simulink model "case5new"  (Simulink 5.0)
settings: Solver=FixedStepDiscrete  SolverMode=SingleTasking  StartTime=0.0  StopTime=1  FixedStep=Ts  RelTol=1e-3  AbsTol=1e-2
PreLoadFcn:
  | assignin('base','Ts',[50e-6])
InitFcn:
  | powericon('psbinitsys',bdroot);
undefined symbols (not defined in the file): D1, Delta, gcbh, powericon, Ts
libraries: powerlib2 x65, powerlib_extras x5
settings Model: Creator=sybille  LastModifiedBy=gnedin pa  ExtModeTrigMode=oneshot  ExtModeArmWhenConnect=off  SaveTime=off  LimitDataPoints=off  UnconnectedInputMsg=none  UnconnectedOutputMsg=none  BlockReductionOpt=off  BooleanDataType=off

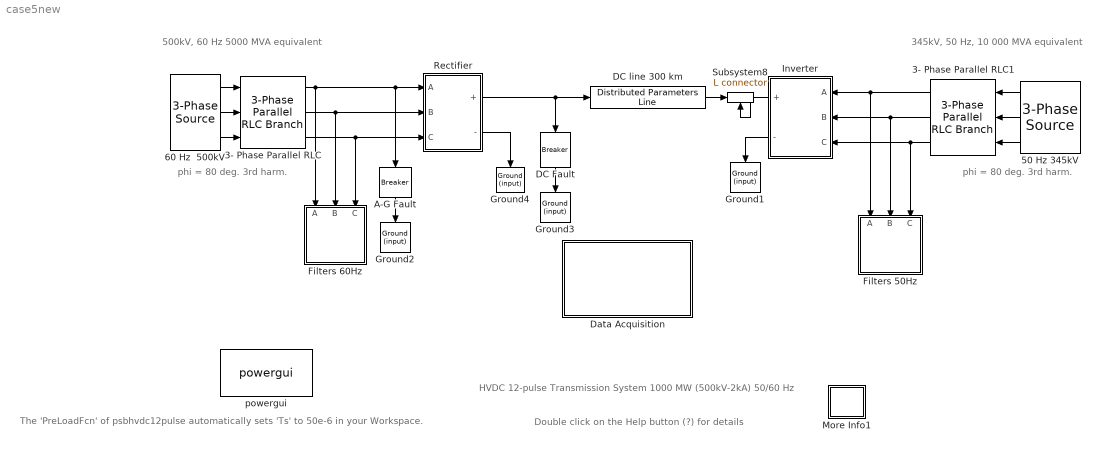
== system case5new ==
  note: phi = 80 deg. 3rd harm.
  note: The 'PreLoadFcn' of psbhvdc12pulse
      | automatically sets 'Ts' to 50e-6 in your Workspace.
  note: Double click on the Help button (?) for details
  note: HVDC 12-pulse Transmission System
      | 1000 MW (500kV-2kA)   50/60 Hz
  note: 500kV, 60 Hz
      |  5000 MVA equivalent
  note: 345kV, 50 Hz,
      | 10 000 MVA equivalent
  note: phi = 80 deg. 3rd harm.
  " 50 Hz 345kV  " : powerlib2/Electrical Sources/3-Phase Source  Tag=PoWeRsYsTeMbLoCk  Orientation=left  V=345e3  Phi=0  F=50  InternalConnection=Yg  RLoff=off  R=0  L=28.0e-3  Psc=0  Vbase=0  XRratio=0  PSBOutputType=111
  " 60 Hz  500kV" : powerlib2/Electrical Sources/3-Phase Source  Tag=PoWeRsYsTeMbLoCk  V=500e3  Phi=0  F=60  InternalConnection=Yg  RLoff=off  R=0  L=98.03e-3  Psc=0  Vbase=0  XRratio=0  PSBOutputType=111
  3- Phase Parallel RLC : powerlib2/Elements/3-Phase Parallel RLC Branch  R=26.07  L=48.86e-3  C=0
  3- Phase Parallel RLC1 : powerlib2/Elements/3-Phase Parallel RLC Branch  Orientation=left  R=6.205  L=13.96e-3  C=0
  A-G Fault : powerlib2/Elements/Breaker  Tag=PoWeRsYsTeMbLoCk  Orientation=down  a=0.01  c=0  rs=inf  cs=inf  times=[ 0.6 0.7]*100  Ts=0  comext=off  mesure=Branch current  PSBOutputType=1
  DC Fault : powerlib2/Elements/Breaker  Tag=PoWeRsYsTeMbLoCk  Orientation=down  a=1  c=0  rs=inf  cs=inf  times=[0.6 0.65]*100  Ts=0  comext=off  mesure=Branch current  PSBOutputType=1
  DC line 300 km : powerlib2/Elements/Distributed Parameters Line  Tag=PoWeRsYsTeMbLoCk  n=1  f=60  r=0.015  l=0.792e-3  c=14.4e-9  lgt=300  x1=[0 0 0 0; 0.0001244 0 0 0; 0.0002488 0 0 0; 0.0003733 0 0 0; 0.0004977 0 0 0; 0.0006221 0 0 0]  x2=[0 0 0 0; 0.0001244 0 0 0; 0.0002488 0 0 0; 0.0003733 0 0 0; 0.0004977 0 0 0; 0.0006221 0 0 0]  x3=[0 0 0 0; 0.0001244 0 0 0; 0.0002488 0 0 0; 0.0003733 0 0 0; 0.0004977 0 0 0; 0.0006221 0 0 0]  x4=[0 0 0 0; 0.0001244 0 0 0; 0.0002488 0 0 0; 0.0003733 0 0 0; 0.0004977 0 0 0; 0.0006221 0 0 0]  x5=0  mesure=None  PSBOutputType=111111111111111111111111111111
  Data Acquisition : Subsystem
      mask Display: disp('Open this block\nto visualize\nrecorded signals')
  Filters 50Hz : Subsystem  Orientation=down
      mask Display: disp('AC filters\n50 Hz\n600 Mvar')
  Filters 60Hz : Subsystem  Orientation=down
      mask Display: disp('AC filters \n60 Hz\n600 Mvar')
  Ground{1..4} (4 alike) : powerlib2/Connectors/Ground (input)  Tag=PoWeRsYsTeMbLoCk  Orientation=down
  Inverter : Subsystem  Orientation=left
  More Info1 : Subsystem
      mask Display: disp('?')
  Rectifier : Subsystem
  Subsystem8 : powerlib2/Connectors/L connector  Tag=PoWeRsYsTeMbLoCk  Orientation=up
  powergui : powerlib2/powergui  Frange=[0:2:500]  Ylog=off  Xlog=on  save=off  variable=ZData  ZoomFFT=on  StartTime=0.0  cycles=1  DisplayStyle=off  fundamental=60  FreqAxis=off  MaxFrequency=1000  frequencyindice=1  frequencyindicesteady=1  RmsSteady=1  display=off  Ts=50e-6  methode=off  frequency=60  echomessages=off
  wires:
  DC Fault/1 -> Ground3/1
  A-G Fault/1 -> Ground2/1
  " 60 Hz  500kV"/1 -> 3- Phase Parallel RLC/1
  " 60 Hz  500kV"/2 -> 3- Phase Parallel RLC/2
  " 60 Hz  500kV"/3 -> 3- Phase Parallel RLC/3
  3- Phase Parallel RLC/2 -> Filters 60Hz/2(B), Rectifier/2(B)
  3- Phase Parallel RLC/1 -> Filters 60Hz/1(A), A-G Fault/1, Rectifier/1(A)
  3- Phase Parallel RLC/3 -> Filters 60Hz/3(C), Rectifier/3(C)
  " 50 Hz 345kV  "/2 -> 3- Phase Parallel RLC1/2
  " 50 Hz 345kV  "/1 -> 3- Phase Parallel RLC1/1
  " 50 Hz 345kV  "/3 -> 3- Phase Parallel RLC1/3
  Rectifier/1("+ ") -> DC line 300 km/1, DC Fault/1
  Rectifier/2(-) -> Ground4/1
  Inverter/2(-) -> Ground1/1
  Inverter/1(+) -> Subsystem8/1
  3- Phase Parallel RLC1/1 -> Filters 50Hz/1(A), Inverter/1(A)
  3- Phase Parallel RLC1/2 -> Filters 50Hz/2(B), Inverter/2(B)
  DC line 300 km/1 -> Subsystem8/Enable
  3- Phase Parallel RLC1/3 -> Filters 50Hz/3(C), Inverter/3(C)

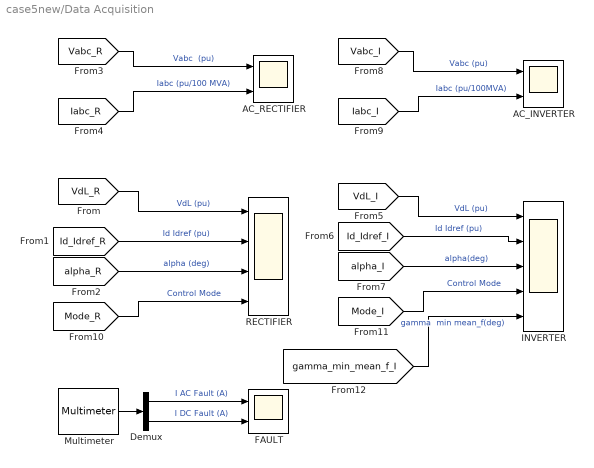
== system case5new/Data Acquisition ==
  AC_INVERTER : Scope  NumInputPorts=2
      settings: TimeRange=0.2008622476996453  YMin=-1.25~-4  YMax=1.25~5  SaveName=ScopeData4  DataFormat=Array  Decimation=Ts  SampleInput=on  SampleTime=Ts
  AC_RECTIFIER : Scope  NumInputPorts=2
      settings: TimeRange=0.2008622476996453  YMin=-1.25~-4  YMax=1.25~5  DataFormat=Array  Decimation=Ts  SampleInput=on  SampleTime=Ts
  Demux : Demux  Outputs=2
  FAULT : Scope  NumInputPorts=2
      settings: TimeRange=0.2008622476996453  YMin=-1.25~-4  YMax=1.25~5  DataFormat=Array  Decimation=Ts  SampleInput=on  SampleTime=Ts
  INVERTER : Scope  NumInputPorts=5
      settings: TimeRange=1  YMin=-0.25~-0.25~75~0~0  YMax=1.25~1.25~175~2~200  SaveName=inv  Decimation=Ts  SampleInput=on  SampleTime=Ts
  Multimeter : powerlib2/Measurements/Multimeter  Tag=PoWeRsYsTeMmEaSuReMeNt  PhasorSimulation=off  OutputType=Magnitude  sel=[11 12]  L=18  Gain=[1 1]  yselected={'Ib: A-G Fault','Ib: DC Fault'};  PSBOutputType=1  PSBequivalent=0  AxesSetting=[0,0.1,-100,100]  Display=0  SavedBlockNames={}
  RECTIFIER : Scope  NumInputPorts=4
      settings: TimeRange=1  YMin=-0.5~-0.5~0~0  YMax=1.5~1.5~100~5  SaveName=rect  Decimation=Ts  SampleInput=on  SampleTime=Ts
  wires:
  [gamma_min_mean_f_I] -> INVERTER/5  "gamma  min mean_f(deg)"
  [Mode_I] -> INVERTER/4  "Control Mode"
  [Mode_R] -> RECTIFIER/4  "Control Mode"
  Demux/2 -> FAULT/2  "I DC Fault (A)"
  Demux/1 -> FAULT/1  "I AC Fault (A)"
  Multimeter/1 -> Demux/1
  [alpha_I] -> INVERTER/3  "alpha(deg)"
  [Id_Idref_I] -> INVERTER/2  "Id Idref (pu)"
  [VdL_I] -> INVERTER/1  "VdL (pu)"
  [Iabc_I] -> AC_INVERTER/2  "Iabc (pu/100MVA)"
  [Vabc_I] -> AC_INVERTER/1  "Vabc (pu)"
  [alpha_R] -> RECTIFIER/3  "alpha (deg)"
  [Id_Idref_R] -> RECTIFIER/2  "Id Idref (pu)"
  [VdL_R] -> RECTIFIER/1  "VdL (pu)"
  [Iabc_R] -> AC_RECTIFIER/2  "Iabc (pu/100 MVA)"
  [Vabc_R] -> AC_RECTIFIER/1  "Vabc  (pu)"

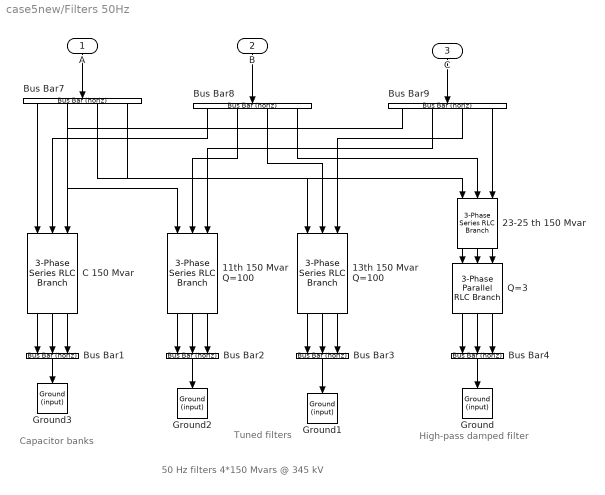
== system case5new/Filters 50Hz ==
  note: 50 Hz filters 4*150 Mvars @ 345 kV
  note: Capacitor banks
  note: Tuned filters
  note: High-pass
      | damped filter
  A : Inport  Orientation=down
  B : Inport  Orientation=down  Port=2
  C : Inport  Orientation=down  Port=3
  " 23-25 th 150 Mvar" : powerlib2/Elements/3-Phase Series RLC Branch   Orientation=down  R=0  L=0  C=4.012e-6
  "11th 150 Mvar Q=100 " : powerlib2/Elements/3-Phase Series RLC Branch   Orientation=down  R=0.7214  L=20.87e-3  C=4.012e-6
  13th 150 Mvar Q=100 : powerlib2/Elements/3-Phase Series RLC Branch   Orientation=down  R=0.6104  L=14.95e-3  C=4.012e-6
  Bus Bar{1..4} (4 alike) : powerlib2/Connectors/Bus Bar (horiz)  Tag=PoWeRsYsTeMbLoCk  Orientation=down  entrees=3  sorties=1  PSBOutputType=1111111111111111111111111111111111111111111111111111111111111111111111111
  Bus Bar7 : powerlib2/Connectors/Bus Bar (horiz)  Tag=PoWeRsYsTeMbLoCk  Orientation=down  entrees=1  sorties=4  PSBOutputType=1111111111111111111111111111111111111111111111111111111111111111111111111
  Bus Bar8 : powerlib2/Connectors/Bus Bar (horiz)  Tag=PoWeRsYsTeMbLoCk  Orientation=down  entrees=1  sorties=4  PSBOutputType=1111111111111111111111111111111111111111111111111111111111111111111111111
  Bus Bar9 : powerlib2/Connectors/Bus Bar (horiz)  Tag=PoWeRsYsTeMbLoCk  Orientation=down  entrees=1  sorties=4  PSBOutputType=1111111111111111111111111111111111111111111111111111111111111111111111111
  C 150 Mvar : powerlib2/Elements/3-Phase Series RLC Branch   Orientation=down  R=0  L=0  C=4.012e-6
  Ground{,1..3} (4 alike) : powerlib2/Connectors/Ground (input)  Tag=PoWeRsYsTeMbLoCk  Orientation=down
  Q=3 : powerlib2/Elements/3-Phase Parallel RLC Branch  Orientation=down  R=99.19  L=4.385e-3  C=0
  wires:
  A/1 -> Bus Bar7/1
  B/1 -> Bus Bar8/1
  C/1 -> Bus Bar9/1
  13th 150 Mvar Q=100/1 -> Bus Bar3/1
  13th 150 Mvar Q=100/2 -> Bus Bar3/2
  13th 150 Mvar Q=100/3 -> Bus Bar3/3
  Q=3/1 -> Bus Bar4/1
  Q=3/2 -> Bus Bar4/2
  Q=3/3 -> Bus Bar4/3
  Bus Bar7/1 -> C 150 Mvar/1
  Bus Bar8/1 -> C 150 Mvar/2
  Bus Bar8/3 -> 13th 150 Mvar Q=100/2
  Bus Bar8/4 -> " 23-25 th 150 Mvar"/2
  Bus Bar7/3 -> 13th 150 Mvar Q=100/1
  Bus Bar7/4 -> " 23-25 th 150 Mvar"/1
  Bus Bar9/1 -> C 150 Mvar/3
  Bus Bar9/3 -> 13th 150 Mvar Q=100/3
  Bus Bar9/4 -> " 23-25 th 150 Mvar"/3
  C 150 Mvar/1 -> Bus Bar1/1
  C 150 Mvar/2 -> Bus Bar1/2
  C 150 Mvar/3 -> Bus Bar1/3
  Bus Bar1/1 -> Ground3/1
  "11th 150 Mvar Q=100 "/1 -> Bus Bar2/1
  "11th 150 Mvar Q=100 "/2 -> Bus Bar2/2
  "11th 150 Mvar Q=100 "/3 -> Bus Bar2/3
  Bus Bar8/2 -> "11th 150 Mvar Q=100 "/2
  Bus Bar7/2 -> "11th 150 Mvar Q=100 "/1
  Bus Bar9/2 -> "11th 150 Mvar Q=100 "/3
  Bus Bar2/1 -> Ground2/1
  Bus Bar3/1 -> Ground1/1
  Bus Bar4/1 -> Ground/1
  " 23-25 th 150 Mvar"/1 -> Q=3/1
  " 23-25 th 150 Mvar"/2 -> Q=3/2
  " 23-25 th 150 Mvar"/3 -> Q=3/3

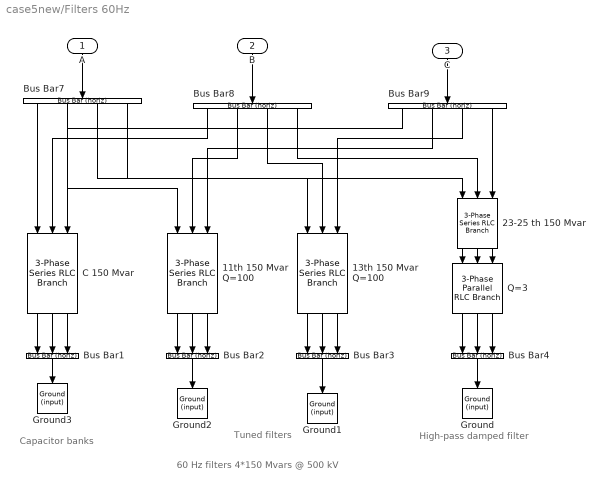
== system case5new/Filters 60Hz ==
  note: 60 Hz filters 4*150 Mvars @ 500 kV
  note: High-pass
      | damped filter
  note: Tuned filters
  note: Capacitor banks
  A : Inport  Orientation=down
  B : Inport  Orientation=down  Port=2
  C : Inport  Orientation=down  Port=3
  " 23-25 th 150 Mvar" : powerlib2/Elements/3-Phase Series RLC Branch   Orientation=down  R=0  L=0  C=1.592e-6
  "11th 150 Mvar Q=100 " : powerlib2/Elements/3-Phase Series RLC Branch   Orientation=down  R=1.515  L=36.53e-3  C=1.592e-6
  13th 150 Mvar Q=100 : powerlib2/Elements/3-Phase Series RLC Branch   Orientation=down  R=1.282  L=26.15e-3  C=1.592e-6
  Bus Bar{1..4} (4 alike) : powerlib2/Connectors/Bus Bar (horiz)  Tag=PoWeRsYsTeMbLoCk  Orientation=down  entrees=3  sorties=1  PSBOutputType=1111111111111111111111111111111111111111111111111111111111111111111111111
  Bus Bar7 : powerlib2/Connectors/Bus Bar (horiz)  Tag=PoWeRsYsTeMbLoCk  Orientation=down  entrees=1  sorties=4  PSBOutputType=1111111111111111111111111111111111111111111111111111111111111111111111111
  Bus Bar8 : powerlib2/Connectors/Bus Bar (horiz)  Tag=PoWeRsYsTeMbLoCk  Orientation=down  entrees=1  sorties=4  PSBOutputType=1111111111111111111111111111111111111111111111111111111111111111111111111
  Bus Bar9 : powerlib2/Connectors/Bus Bar (horiz)  Tag=PoWeRsYsTeMbLoCk  Orientation=down  entrees=1  sorties=4  PSBOutputType=1111111111111111111111111111111111111111111111111111111111111111111111111
  C 150 Mvar : powerlib2/Elements/3-Phase Series RLC Branch   Orientation=down  R=0  L=0  C=1.592e-6
  Ground{,1..3} (4 alike) : powerlib2/Connectors/Ground (input)  Tag=PoWeRsYsTeMbLoCk  Orientation=down
  Q=3 : powerlib2/Elements/3-Phase Parallel RLC Branch  Orientation=down  R=208.3  L=7.673e-3  C=0
  wires:
  " 23-25 th 150 Mvar"/3 -> Q=3/3
  " 23-25 th 150 Mvar"/2 -> Q=3/2
  " 23-25 th 150 Mvar"/1 -> Q=3/1
  Bus Bar4/1 -> Ground/1
  Bus Bar3/1 -> Ground1/1
  Bus Bar2/1 -> Ground2/1
  Bus Bar9/2 -> "11th 150 Mvar Q=100 "/3
  Bus Bar7/2 -> "11th 150 Mvar Q=100 "/1
  Bus Bar8/2 -> "11th 150 Mvar Q=100 "/2
  "11th 150 Mvar Q=100 "/3 -> Bus Bar2/3
  "11th 150 Mvar Q=100 "/2 -> Bus Bar2/2
  "11th 150 Mvar Q=100 "/1 -> Bus Bar2/1
  Bus Bar1/1 -> Ground3/1
  C 150 Mvar/3 -> Bus Bar1/3
  C 150 Mvar/2 -> Bus Bar1/2
  C 150 Mvar/1 -> Bus Bar1/1
  Bus Bar9/4 -> " 23-25 th 150 Mvar"/3
  Bus Bar9/3 -> 13th 150 Mvar Q=100/3
  Bus Bar9/1 -> C 150 Mvar/3
  Bus Bar7/4 -> " 23-25 th 150 Mvar"/1
  Bus Bar7/3 -> 13th 150 Mvar Q=100/1
  Bus Bar8/4 -> " 23-25 th 150 Mvar"/2
  Bus Bar8/3 -> 13th 150 Mvar Q=100/2
  Bus Bar8/1 -> C 150 Mvar/2
  Bus Bar7/1 -> C 150 Mvar/1
  Q=3/3 -> Bus Bar4/3
  Q=3/2 -> Bus Bar4/2
  Q=3/1 -> Bus Bar4/1
  13th 150 Mvar Q=100/3 -> Bus Bar3/3
  13th 150 Mvar Q=100/2 -> Bus Bar3/2
  13th 150 Mvar Q=100/1 -> Bus Bar3/1
  C/1 -> Bus Bar9/1
  B/1 -> Bus Bar8/1
  A/1 -> Bus Bar7/1

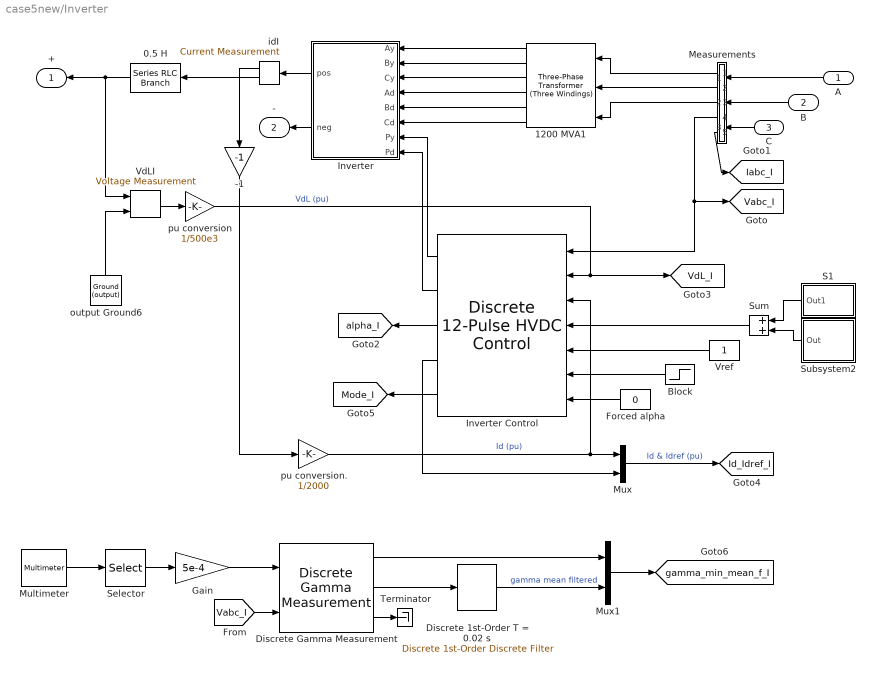
== system case5new/Inverter ==
  A : Inport  Orientation=left
  B : Inport  Orientation=left  Port=2
  C : Inport  Orientation=left  Port=3
  -1 : Gain  Orientation=down  Gain=-1  SaturateOnIntegerOverflow=on
  0.5 H : powerlib2/Elements/Series RLC Branch  Tag=PoWeRsYsTeMbLoCk  Orientation=left  a=1  b=0.5  c=inf  mesure=None  PSBOutputType=1
  1200 MVA1 : powerlib2/Elements/Three-Phase Transformer (Three Windings)  Tag=PoWeRsYsTeMbLoCk  Orientation=left  confi=ABC as input terminals  nom=[ 1200e6 , 50 ]  ydw1=Yg  w1="[ 345e3*0.96 0.0025  0 ]"  ydw2=Y  w2="[ 200e3  0.0025 0.24]"  ydw3=Delta (D1)  w3=[ 200e3 0.0025 0.24 ]  ynsat=off  rmag=500  lm=500  sat=[0 0; 1 1.2; 2 1.1]  hyst=off  matfile='hysteresis'  sif=off  ifl=[0.8 -0.8 0.7]  initialslopes=[+1 +1 +1]  mesure=None  PSBOutputType=111111
  Block : Step  Orientation=left  Time=0.02  Before=1  After=0  SampleTime=0
  Discrete 1st-Order T = 0.02 s : powerlib_extras/Discrete  Control Blocks/Discrete 1st-Order Discrete Filter  FilterType=Lowpass  Tc=1/50  Ts=Ts  Initialize=off  Vac_Init=[0.8 -25 60]  Vdc_Init=-0.4  PlotResponse=off  param1=[1 500 0.1]
  Discrete Gamma Measurement : powerlib_extras/Discrete  Control Blocks/Discrete Gamma Measurement  f0=50  dt=Ts
  Forced alpha : Constant  Orientation=left  Value=0
  Gain : Gain  Gain=5e-4  SaturateOnIntegerOverflow=on
  Inverter : Subsystem  Orientation=left
      mask Display: plot(0,0,100,100,[30 70 50 30 ], [60 60 40 60], [50 50], [25 40], [50 50], [ 60 75], [30 70], [40 40], [50 60 70], [40 30 30]);
  Inverter Control : powerlib_extras/Discrete  Control Blocks/Discrete 12-Pulse HVDC Control   Orientation=left  Mode=Inverter  f0Pw=[50 101.5]  XPILimR=[165, 5]  XLinR=[60, 20]  XPILimI=[165, 92]  XLinI="[160,  120]"  Xmarg="[0.1,  0.05]"  XKPI_I=[45, 4500, 90]  XKPI_V="[35, 2250,  90]"  T1_I=0.3e-3  XT_V=[10e-3 , 0.1e-3]  BP=25  Xvdcol=[0.6, 0.18, 0.30, 0.1, 0.080]  alpha_const=off  alpha_fix=165  pas=Ts
  Measurements : Subsystem  Tag=PoWeRsYsTeMmEaSuReMeNt  Orientation=left  AncestorBlock=powerlib2/Measurements/Three-Phase V-I Measurement  LoadFcn=powericon('psbloadfunction',gcbh,'3-Phase VI Measurement','');  InitFcn=powericon('checksum',bdroot)  mask(3-Phase VI Measurement){VChoice=phase-to-ground, ualv=off, labelV=V1, Vpu=on, Vbase=345e3, IChoice=yes, ualc=off, labelC=I1, Ppu=on, Pbase=100e6, OutputType=Magnitude, PhasorSimulation=off, PSBequivalent=0, PSBOutputType=11100}
      mask prompts: VChoice "Voltage measurement"; ualv "Use a label"; labelV "Signal label  (use a From block to collect signal)"; Vpu "Voltage  in pu"; Vbase "Base voltage (Vrms phase-phase) :"; IChoice "Current measurement"; ualc "Use a label"; labelC "Signal label  (use a From block to collect signal)"; Ppu "Currents in pu"; Pbase "Base power ( VA 3 phase)"; OutputType "Output signal :"; PhasorSimulation "Phasor simulation"; PSBequivalent "Equivalent circuit"
      mask help:
      | This block is used to measure three-phase voltages and currents in a circuit. When connected in series with a three-phase element, it return the three phase-to-ground voltages and line currents.
      |
      | The block can output the voltages and currents in per unit values or in volts and amperes. Check the appropriate boxes if you want to output the voltages and currents  in pu
      mask init:
      | powericon('psbcallbacks',gcb,'Three-phase measurements',4);
      | if  Vpu
      |     xKv=1/(Vbase/sqrt(3)*sqrt(2));
      | else
      |     xKv=1;
      | end
      | if  Ppu
      |     xKi=1/(Pbase/Vbase/sqrt(3)*sqrt(2));
      | else
      |     xKi=1;
      | end
      | switch OutputType
      | case 1
      |     OutputSelection  = [1:6];
      |     PhasorModeV = [1:3];
      |     NormalModeV = [7:9];
      |     PhasorModeI = [4:6];
      |     NormalModeI = [10:12];
      |     Kv = xKv;
      |     Ki = xKi;
      | case 2
      |     OutputSelection = [7,13,8,14,9,15,10,16,11,17,12,18];
      |     PhasorModeV = [1:6];
      |     NormalModeV = [13:15];
      |     PhasorModeI = [7:12];
      |     NormalModeI = [16:18];
      |     Kv = xKv;
      |     Ki = xKi;
      | case 3
      |     OutputSelection = [13,19,14,20,15,21,16,22,17,23,18,24];
      |     PhasorModeV = [1:6];
      |     NormalModeV = [13:15];
      |     PhasorModeI = [7:12];
      |     NormalModeI = [16:18];
      |     Kv = [xKv 1 xKv 1 xKv 1];
      |     Ki = [xKi 1 xKi 1 xKi 1];
      | case 4
      |     OutputSelection  = [19:24];
      |     PhasorModeV = [1:3];
      |     NormalModeV = [7:9];
      |     PhasorModeI = [4:6];
      |     NormalModeI = [10:12];
      |     Kv = xKv;
      |     Ki = xKi;
      | end
      | if PhasorSimulation
      |     SelectionModeV = PhasorModeV;
      |     SelectionModeI = PhasorModeI;
      | else
      |     SelectionModeV = NormalModeV;
      |     SelectionModeI = NormalModeI;
      |     Kv = xKv;
      |     Ki = xKi;
      | end
      settings: CopyFcn=powericon('psbloadfunction',gcbh,'3-Phase VI Measurement','VerifyPhasor');  CloseFcn=%3phaseVImeasurement
      mask Help: web(psbhelp)
      mask StyleString: popup(no|phase-to-ground|phase-to-phase),checkbox,edit,checkbox,edit,popup(no|yes),checkbox,edit,checkbox,edit,popup(Complex|Real-Imag|Magnitude-Angle|Magnitude),checkbox,edit,edit
      mask CallbackString: powericon('psbcallbacks',gcb,'Three-phase measurements',2);|powericon('psbcallbacks',gcb,'Three-phase measurements',2);||powericon('psbcallbacks',gcb,'Three-phase measurements',2);||powericon('psbcallbacks',gcb,'Three-phase measurements',2);|powericon('psbcallbacks',gcb,'Three-phase measurements',2);||powericon('psbcallbacks',gcb,'Three-phase measurements',4);|||||
  Multimeter : powerlib2/Measurements/Multimeter  Tag=PoWeRsYsTeMmEaSuReMeNt  PhasorSimulation=off  OutputType=Magnitude  sel=[13 14 15 16 17 18 1]  L=18  Gain=[1 1 1 1 1 1 1]  yselected={'Isw1: Inverter/Inverter/Universal Bridge','Isw2: Inverter/Inverter/Universal Bridge','Isw3: Inverter/Inverter/Universal Bridge','Isw4: Inverter/Inverter/Universal Bridge','Isw5: Inverter/Inverter/Universal Bridge','Isw6: Inverter/Inverter/Universal Bridge','Usw1: Inverter/Inverter/Universal Bridge'};  PSBOutputType=1  PSBequivalent=0  AxesSetting=[0,0.1,-100,100]  Display=0  SavedBlockNames=-11
  Mux : Mux  Inputs=2
  Mux1 : Mux  Inputs=2
  S1 : Subsystem  Orientation=left  mask(RAMPING UNIT){F_up=1.0, up_slope=1.0/0.4, T_up=0.02, F_down=0., down_slope=-1, T_down=100}
      mask prompts: F_up "Final Up Value (pu):"; up_slope "Up Slope (pu/s):"; T_up "Start Up Time (s):"; F_down "Final Down Value (pu):"; down_slope "Down Slope (pu/s):"; T_down "Start Down Time (s):"
      mask init:
      | T_up_final      =  T_up + F_up/up_slope;
      | T_down_final =   T_down + (F_down-F_up)/down_slope;
      | T_ramp  = [0, T_up, T_up_final,  T_down,  T_down_final, 9999]';
      | U_ramp = [0, 0 , F_up,  F_up,  F_down,  F_down]';
      mask Display: disp('Ramping\n Unit')
  Selector : Selector  Elements=[1 2 3 4 5 6]  InputPortWidth=7
  Subsystem2 : Subsystem  Orientation=left
      mask Display: disp('Step Up\n & Down')
  Sum : Sum  Orientation=left  SaturateOnIntegerOverflow=on  InputSameDT=on
  Terminator : Terminator
  VdLI : powerlib2/Measurements/Voltage Measurement  Tag=PoWeRsYsTeMmEaSuReMeNt  PhasorSimulation=off  OutputType=Magnitude  PSBOutputType=0  PSBequivalent=0
  Vref : Constant  Orientation=left
  idI : powerlib2/Measurements/Current Measurement  Tag=PoWeRsYsTeMmEaSuReMeNt  Orientation=left  PhasorSimulation=off  OutputType=Magnitude  PSBOutputType=01  PSBequivalent=0
  output Ground6 : powerlib2/Connectors/Ground (output)  Tag=PoWeRsYsTeMbLoCk  Orientation=up  PSBOutputType=1
  pu conversion : Gain  Gain=1/500e3  SaturateOnIntegerOverflow=on
  pu conversion. : Gain  Gain=1/2000  SaturateOnIntegerOverflow=on
  + : Outport  Orientation=left
  - : Outport  Orientation=left  Port=2
  tag scope: Iabc_I=global, Id_Idref_I=global, Mode_I=global, Vabc_I=global, VdL_I=global, alpha_I=global, gamma_min_mean_f_I=global
  wires:
  Discrete Gamma Measurement/3 -> Terminator/1
  Selector/1 -> Gain/1
  Discrete 1st-Order T = 0.02 s/1 -> Mux1/2  "gamma mean filtered"
  Mux1/1 -> [gamma_min_mean_f_I]
  Subsystem2/1(Out) -> Sum/2
  Discrete Gamma Measurement/2 -> Discrete 1st-Order T = 0.02 s/1
  Discrete Gamma Measurement/1 -> Mux1/1
  [Vabc_I] -> Discrete Gamma Measurement/2
  Gain/1 -> Discrete Gamma Measurement/1
  Multimeter/1 -> Selector/1
  Inverter Control/5 -> [Mode_I]
  -1/1 -> pu conversion./1
  Inverter/2(neg) -> -/1
  Measurements/3("C ") -> 1200 MVA1/3
  Measurements/1("A ") -> 1200 MVA1/1
  output Ground6/1 -> VdLI/2
  pu conversion./1 -> Inverter Control/3, Mux/1  "Id (pu)"
  0.5 H/1 -> VdLI/1, +/1
  Measurements/5(Iabc) -> [Iabc_I]
  S1/1(Out1) -> Sum/1
  idI/2 -> 0.5 H/1
  C/1 -> Measurements/3(C)
  B/1 -> Measurements/2(B)
  Measurements/2("B ") -> 1200 MVA1/2
  A/1 -> Measurements/1(A)
  Block/1 -> Inverter Control/6
  Sum/1 -> Inverter Control/4
  Measurements/4(Vabc) -> Inverter Control/1, [Vabc_I]
  VdLI/1 -> pu conversion/1
  Forced alpha/1 -> Inverter Control/7
  Vref/1 -> Inverter Control/5
  Inverter Control/4 -> Mux/2
  pu conversion/1 -> [VdL_I], Inverter Control/2  "VdL (pu)"
  idI/1 -> -1/1
  Mux/1 -> [Id_Idref_I]  "Id & Idref (pu)"
  Inverter Control/3 -> [alpha_I]
  Inverter Control/1 -> Inverter/7(Py)
  Inverter Control/2 -> Inverter/8(Pd)
  1200 MVA1/6 -> Inverter/6(Cd)
  1200 MVA1/5 -> Inverter/5(Bd)
  1200 MVA1/4 -> Inverter/4(Ad)
  1200 MVA1/3 -> Inverter/3(Cy)
  1200 MVA1/2 -> Inverter/2(By)
  1200 MVA1/1 -> Inverter/1(Ay)
  Inverter/1(pos) -> idI/1

== system case5new/More Info1 ==
  note: In the DC Fault block and Forced Delay Timer blocks, change the multiplication factor of 1 in the Transition Times to 100,
      | so that the DC fault is now eliminated.  In the AC Fault block, change the multiplication factor in the Transition Times to 1,
      | so that a 6 cycles line-to-ground fault is now applied at the rectifier. Restart the simulation.
      |
      | Notice the 120 Hz oscillations in the DC voltage and currents during the fault. When the fault is cleared at t = 0.7 s,
      | the VDCOL operates and reduces the reference current to 0.3 pu. The system recovers in approximately 0.4 s after fault clearing.
  note: AC line-to-ground fault
  note: In order to eliminate the step disturbance applied on the reference current, disconnect the Step Up & Down blocks in the Rectifier and Inverter subsystems.
      | Change to 1 the "100" multiplication factor  in the Transition times of the DC Fault breaker and of the Forced Delay Timer block.
      | so that a fault is now applied at t = 0.6s. Open the FAULT scope to observe the DC fault current. Restart the simulation.
      |
      | At fault application the DC current quickly increases to 2.3 pu and the DC voltage falls to zero at the rectifier.
      | This DC voltages drop is seen by the Voltage Dependant Currrent Order Limiter (VDCOL) which reduces the reference current to 0.3 pu at the rectifier.
      | A DC current still continues to circulate in the fault. Then, a t = 0.65 s, the rectifier alpha firing angle is forced to 165 degrees by the protection systems (not simulated).
      | The rectifier now operates in inverter mode. The DC line voltage becomes negative and the energy stored in the line is returned to the AC network,
      | causing rapid extinction of the fault current at its next zero-crossing. Then, alpha is released at t = 0.7 s and the normal DC voltage and current
      | recover in approcxximately 0.3 s.
  note: DC line fault
  note: Start-up
  note: DEMONSTRATION
  note: A 1000 MW (500 kV, 2kA) DC linterconnexion is used to transmit power from a 500 kV, 5000 MVA, 60 Hz network.
      | to a  345 kV, 10 000 MVA, 50 Hz network.
      |
      | The rectifier and the inverter  are 12-pulse converters using  two 6-pulse thyristor briges connected in series.
      | The converter and the inverter are interconnected through a 300 km distributed parameter line through 0.5 H smoothing reactors.
      | The transformers are modeled with Universal Transformer blocks.
      | The transformer tap changers are not simulated and  fixed taps are assumed. Open the two transformer blocks in the Rectifier and Inverter subsystems
      | to see the factors applied on the primary voltage: 0.90 on rectifier side and 0.96 on inverter side. Reactive power required by the converters is provided
      | by a set of capacitor banks plus 11th, 13th and  high pass filters for a total of  600 Mvar on each side.
      | Two circuit breakers are used to apply faults on the rectifier AC and DC sides.
      |
      | The rectifier and inverter control systems use the  Discrete 12-pulse HVDC Control block of the Extras/Control library.
      | The power system and the control system are both  discretized for a sample time = Ts.
      | A description of the control systems is provided in the HVDC Transmission System Case Study of the User's Manual.
  note: Steady-state and transient performance of a 12-pulse,
      | 1000 MW (500 kV-2kA) 50/60 Hz HVDC transmission system
  note: CIRCUIT DESCRIPTION
  note: Notice that the "PreLoadFcn" function of the model  automatically sets Ts = 50e-6 in your Matlab workspace.
      | The system is programmed to start and  reach a steady state.  Then, a step is applied on the reference current to observe the dynamic response
      | of the regulators. Start the simulation and open the 'Data Acquisition' block to visualize  signals displayed on RECTIFIER and  INVERTER scopes.
  note: At  0.6 seconds, a 0.2 pu step is applied on the reference current (decrease from 1 pu  to 0.8 pu ).
      | At 0.75 seconds, another step is applied to set the reference back to 1 pu.
      | Observe the response of the current regulator.  It stabilizes in  approximately 0.05 seconds.
  note: Step reponse of regulators
  note: S. Casoria (Hydro-Québec)
  note: The reference current is ramped from zero to 1 pu (2kA) in 0.4 s. The DC current and voltages start from zero and reach steady-state
      | in approximately 0.5 s. At the end, the RECTIFIER controls the current and the INVERTER controls the voltage. Trace 1 of  the RECTIFIER and INVERTER scopes
      | shows the DC line voltage (1pu = 500 kV). Trace 2 shows the the reference current and the measured Id current (1pu = 2kA). In steady-state, the alpha firing
      | angles (trace 3) are 18 degrees and 142 degrees respectively on the RECTIFIER and INVERTER sides. The exctinction angle gamma (minimum and mean values) is
      | measured at the INVERTER  and shown in trace 4. In steady-state, the mean value is between 24 and 25 degrees. The gamma measurement block is found in the
      | Discrete Control Blocks of the Extras librairy. The control mode of operation (number between 0 to 5: 0- blocked; 1- Current control; 2- Voltage control;
      | 3- Alpha minimum limitation;  4- Alpha maximum limitation; 5- Forced or constant alpha) is shown in trace 4.

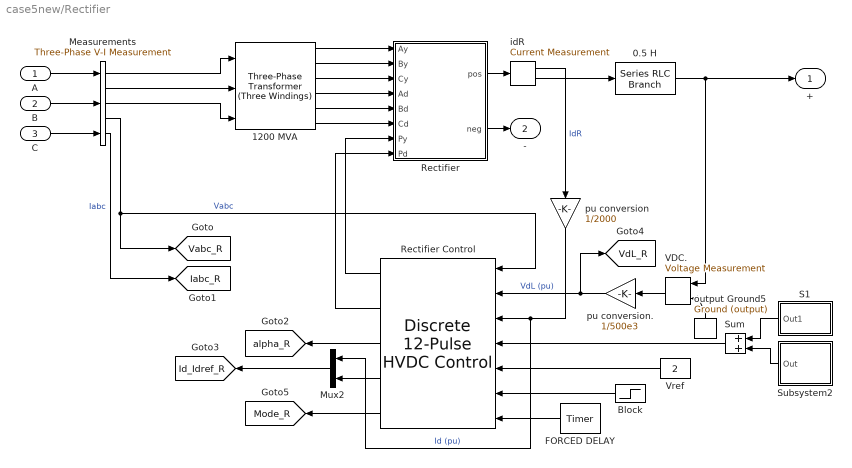
== system case5new/Rectifier ==
  A : Inport
  B : Inport  Port=2
  C : Inport  Port=3
  "0.5 H " : powerlib2/Elements/Series RLC Branch  Tag=PoWeRsYsTeMbLoCk  a=1  b=0.5  c=inf  mesure=None  PSBOutputType=1
  1200 MVA : powerlib2/Elements/Three-Phase Transformer (Three Windings)  Tag=PoWeRsYsTeMbLoCk  confi=ABC as input terminals  nom=[ 1200e6 , 60 ]  ydw1=Yg  w1="[ 500e3*0.9 0.0025  0 ]"  ydw2=Y  w2=[ 200e3 0.0025 0.24]  ydw3=Delta (D1)  w3=[ 200e3 0.0025 0.24 ]  ynsat=off  rmag=500  lm=500  sat=[0 0; 1 1.2; 2 1.1]  hyst=off  matfile='hysteresis'  sif=off  ifl=[0.8 -0.8 0.7]  initialslopes=[+1 +1 +1]  mesure=None  PSBOutputType=111111
  Block : Step  Orientation=left  Time=0.02  Before=1  After=0  SampleTime=0
  FORCED DELAY : powerlib_extras/Control  Blocks/Timer  Orientation=left  t=[0.65 0.7]*100  e=[ 1 0 ]
  Measurements : powerlib2/Measurements/Three-Phase V-I Measurement  Tag=PoWeRsYsTeMmEaSuReMeNt  VChoice=phase-to-ground  ualv=off  labelV=V1  Vpu=on  Vbase=500e3  IChoice=yes  ualc=off  labelC=I1  Ppu=on  Pbase=100e6  OutputType=Magnitude  PhasorSimulation=off  PSBequivalent=0  PSBOutputType=11100
  Mux2 : Mux  Orientation=left  Inputs=2
  Rectifier : Subsystem
      mask Display: plot(0,0,100,100,[30 70 50 30 ], [40 40 60 40], [50 50], [25 40], [50 50], [ 60 75], [30 70], [60 60], [50 40 30], [60 70 70]);
  Rectifier Control : powerlib_extras/Discrete  Control Blocks/Discrete 12-Pulse HVDC Control   Orientation=left  Mode=Rectifier  f0Pw=[60 101.5]  XPILimR=[165, 5]  XLinR=[60, 20]  XPILimI=[165, 92]  XLinI="[160,  120]"  Xmarg="[0.1,  0.05]"  XKPI_I=[45, 4500, 90]  XKPI_V=[35, 2250, 90]  T1_I=0.3e-3  XT_V=[10e-3 , 0.1e-3]  BP=30  Xvdcol=[0.6, 0.18, 0.30, 0.1, 0.080]  alpha_const=off  alpha_fix=165  pas=Ts
  S1 : Subsystem  Orientation=left  mask(RAMPING UNIT){F_up=1.0, up_slope=1.0/0.4, T_up=0.02, F_down=0., down_slope=-1, T_down=100}
      mask prompts: F_up "Final Up Value (pu):"; up_slope "Up Slope (pu/s):"; T_up "Start Up Time (s):"; F_down "Final Down Value (pu):"; down_slope "Down Slope (pu/s):"; T_down "Start Down Time (s):"
      mask init: same as case5new/Inverter/S1
      mask Display: disp('Ramping\n Unit')
  Subsystem2 : Subsystem  Orientation=left
      mask Display: disp('Step Up\n & Down')
  Sum : Sum  Orientation=left  SaturateOnIntegerOverflow=on  InputSameDT=on
  VDC. : powerlib2/Measurements/Voltage Measurement  Tag=PoWeRsYsTeMmEaSuReMeNt  Orientation=left  PhasorSimulation=off  OutputType=Magnitude  PSBOutputType=0  PSBequivalent=0
  Vref : Constant  Orientation=left  Value=2
  idR : powerlib2/Measurements/Current Measurement  Tag=PoWeRsYsTeMmEaSuReMeNt  PhasorSimulation=off  OutputType=Magnitude  PSBOutputType=01  PSBequivalent=0
  output Ground5 : powerlib2/Connectors/Ground (output)  Tag=PoWeRsYsTeMbLoCk  Orientation=up  PSBOutputType=1
  pu conversion : Gain  Orientation=down  Gain=1/2000  SaturateOnIntegerOverflow=on
  pu conversion. : Gain  Orientation=left  Gain=1/500e3  SaturateOnIntegerOverflow=on
  "+ " : Outport
  - : Outport  Port=2
  tag scope: Iabc_R=global, Id_Idref_R=global, Mode_R=global, Vabc_R=global, VdL_R=global, alpha_R=global
  wires:
  Subsystem2/1(Out) -> Sum/2
  Rectifier Control/5 -> [Mode_R]
  Rectifier/2(neg) -> -/1
  VDC./1 -> pu conversion./1
  output Ground5/1 -> VDC./2
  "0.5 H "/1 -> VDC./1, "+ "/1
  Rectifier Control/3 -> [alpha_R]
  Block/1 -> Rectifier Control/6
  S1/1(Out1) -> Sum/1
  Sum/1 -> Rectifier Control/4
  C/1 -> Measurements/3
  B/1 -> Measurements/2
  idR/2 -> "0.5 H "/1
  A/1 -> Measurements/1
  Measurements/4 -> [Vabc_R], Rectifier Control/1  "Vabc"
  FORCED DELAY/1 -> Rectifier Control/7
  Rectifier/1(pos) -> idR/1
  Rectifier Control/4 -> Mux2/2
  pu conversion/1 -> Mux2/1, Rectifier Control/3  "Id (pu)"
  Mux2/1 -> [Id_Idref_R]
  pu conversion./1 -> [VdL_R], Rectifier Control/2  "VdL (pu)"
  idR/1 -> pu conversion/1  "IdR"
  Rectifier Control/2 -> Rectifier/8(Pd)
  Rectifier Control/1 -> Rectifier/7(Py)
  Vref/1 -> Rectifier Control/5
  Measurements/5 -> [Iabc_R]  "Iabc"
  Measurements/1 -> 1200 MVA/1
  1200 MVA/3 -> Rectifier/3(Cy)
  1200 MVA/2 -> Rectifier/2(By)
  1200 MVA/1 -> Rectifier/1(Ay)
  1200 MVA/5 -> Rectifier/5(Bd)
  1200 MVA/6 -> Rectifier/6(Cd)
  1200 MVA/4 -> Rectifier/4(Ad)
  Measurements/3 -> 1200 MVA/3
  Measurements/2 -> 1200 MVA/2

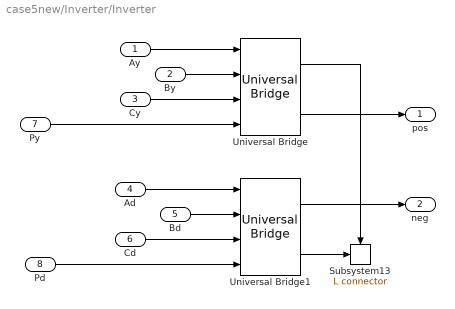
== system case5new/Inverter/Inverter ==
  Ay : Inport
  By : Inport  Port=2
  Cy : Inport  Port=3
  Ad : Inport  Port=4
  Bd : Inport  Port=5
  Cd : Inport  Port=6
  Py : Inport  Port=7
  Pd : Inport  Port=8
  Subsystem13 : powerlib2/Connectors/L connector  Tag=PoWeRsYsTeMbLoCk
  Universal Bridge : powerlib2/Power Electronics/Universal Bridge  Tag=PoWeRsYsTeMbLoCk  arms=3  confi=ABC as input terminals  injcc=2000  cf=0.1e-6  device=Thyristors  Ron=1e-3  Lon=0  VFs="[  0.8  0.8  ]"  Vf=0  gtoparameters=[ 10e-6 , 20e-6 ]  igbtparameters=[ 1e-6 , 2e-6 ]  mesure=All voltages and currents  PSBOutputType=111
  Universal Bridge1 : powerlib2/Power Electronics/Universal Bridge  Tag=PoWeRsYsTeMbLoCk  arms=3  confi=ABC as input terminals  injcc=2000  cf=0.1e-6  device=Thyristors  Ron=1e-3  Lon=0  VFs="[  0.8  0.8  ]"  Vf=0  gtoparameters=[ 10e-6 , 20e-6 ]  igbtparameters=[ 1e-6 , 2e-6 ]  mesure=None  PSBOutputType=111
  pos : Outport
  neg : Outport  Port=2
  wires:
  Universal Bridge1/1 -> neg/1
  Universal Bridge/2 -> pos/1
  Universal Bridge1/2 -> Subsystem13/1
  Universal Bridge/1 -> Subsystem13/Enable
  Ay/1 -> Universal Bridge/1
  By/1 -> Universal Bridge/2
  Cy/1 -> Universal Bridge/3
  Ad/1 -> Universal Bridge1/1
  Bd/1 -> Universal Bridge1/2
  Cd/1 -> Universal Bridge1/3
  Py/1 -> Universal Bridge/4
  Pd/1 -> Universal Bridge1/4

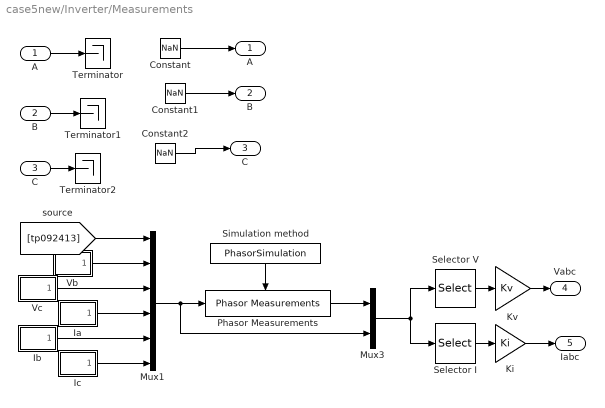
== system case5new/Inverter/Measurements ==
  A : Inport
  B : Inport  Port=2
  C : Inport  Port=3
  Constant : Constant  Value=NaN
  Constant1 : Constant  Value=NaN
  Constant2 : Constant  Value=NaN
  Ia : Subsystem  AncestorBlock=powerlib2/Measurements/Three-Phase V-I Measurement/Ia
  Ib : Subsystem  AncestorBlock=powerlib2/Measurements/Three-Phase V-I Measurement/Ib
  Ic : Subsystem  AncestorBlock=powerlib2/Measurements/Three-Phase V-I Measurement/Ic
  Ki : Gain  Gain=Ki  SaturateOnIntegerOverflow=on
  Kv : Gain  Gain=Kv  SaturateOnIntegerOverflow=on
  Mux1 : Mux  Inputs=6
  Mux3 : Mux  Inputs=2
  Phasor Measurements : powerlib2/Measurements/Three-Phase V-I Measurement/Phasor Measurements  TreatAsAtomicUnit=on  SimViewingDevice=off  DataTypeOverride=UseLocalSettings  MinMaxOverflowLogging=UseLocalSettings
      settings: Permissions=ReadWrite  RTWFcnNameOpts=Auto  RTWFileNameOpts=Auto
  Selector I : Selector  Elements=SelectionModeI  InputPortWidth=length(OutputSelection)+6
  Selector V : Selector  Elements=SelectionModeV  InputPortWidth=length(OutputSelection)+6
  Simulation method : Constant  Orientation=down  Value=PhasorSimulation
  Terminator : Terminator
  Terminator1 : Terminator
  Terminator2 : Terminator
  Vb : Subsystem  AncestorBlock=powerlib2/Measurements/Three-Phase V-I Measurement/Vb
  Vc : Subsystem  AncestorBlock=powerlib2/Measurements/Three-Phase V-I Measurement/Vc
  "A " : Outport
  "B " : Outport  Port=2
  "C " : Outport  Port=3
  Vabc : Outport  Port=4
  Iabc : Outport  Port=5
  wires:
  A/1 -> Terminator/1
  B/1 -> Terminator1/1
  C/1 -> Terminator2/1
  Constant/1 -> "A "/1
  Constant1/1 -> "B "/1
  Constant2/1 -> "C "/1
  Kv/1 -> Vabc/1
  Ki/1 -> Iabc/1
  Selector V/1 -> Kv/1
  Selector I/1 -> Ki/1
  Mux3/1 -> Selector I/1, Selector V/1
  Phasor Measurements/1 -> Mux3/1
  Simulation method/1 -> Phasor Measurements/Enable
  Mux1/1 -> Mux3/2, Phasor Measurements/1
  [tp092413] -> Mux1/1
  Vb/1(Out1) -> Mux1/2
  Vc/1(Out1) -> Mux1/3
  Ia/1(Out1) -> Mux1/4
  Ib/1(Out1) -> Mux1/5
  Ic/1(Out1) -> Mux1/6

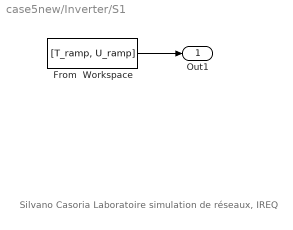
== system case5new/Inverter/S1 ==
  note: Silvano Casoria
      | Laboratoire simulation de réseaux, IREQ
  From  Workspace : FromWorkspace  VariableName="[T_ramp,  U_ramp]"  SampleTime=0
  Out1 : Outport  InitialOutput=0
  wires:
  From  Workspace/1 -> Out1/1

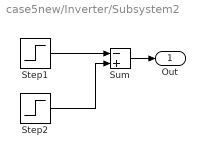
== system case5new/Inverter/Subsystem2 ==
  Step1 : Step  Time=0.6  After=0.2  SampleTime=0
  Step2 : Step  Time=0.75  After=0.2  SampleTime=0
  Sum : Sum  Inputs=-+  SaturateOnIntegerOverflow=on  InputSameDT=on
  Out : Outport
  wires:
  Sum/1 -> Out/1
  Step2/1 -> Sum/2
  Step1/1 -> Sum/1

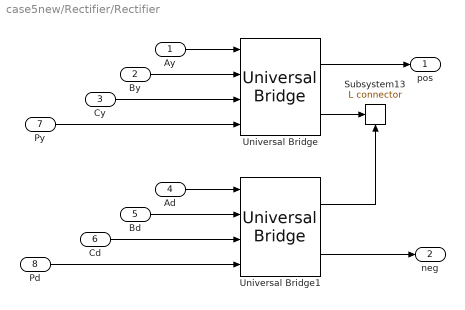
== system case5new/Rectifier/Rectifier ==
  Ay : Inport
  By : Inport  Port=2
  Cy : Inport  Port=3
  Ad : Inport  Port=4
  Bd : Inport  Port=5
  Cd : Inport  Port=6
  Py : Inport  Port=7
  Pd : Inport  Port=8
  Subsystem13 : powerlib2/Connectors/L connector  Tag=PoWeRsYsTeMbLoCk  Orientation=up
  Universal Bridge : powerlib2/Power Electronics/Universal Bridge  Tag=PoWeRsYsTeMbLoCk  arms=3  confi=ABC as input terminals  injcc=2000  cf=0.1e-6  device=Thyristors  Ron=1e-3  Lon=0  VFs="[  0.8  0.8  ]"  Vf=0  gtoparameters=[ 10e-6 , 20e-6 ]  igbtparameters=[ 1e-6 , 2e-6 ]  mesure=None  PSBOutputType=111
  Universal Bridge1 : powerlib2/Power Electronics/Universal Bridge  Tag=PoWeRsYsTeMbLoCk  arms=3  confi=ABC as input terminals  injcc=2000  cf=0.1e-6  device=Thyristors  Ron=1e-3  Lon=0  VFs="[  0.8  0.8  ]"  Vf=0  gtoparameters=[ 10e-6 , 20e-6 ]  igbtparameters=[ 1e-6 , 2e-6 ]  mesure=None  PSBOutputType=111
  pos : Outport
  neg : Outport  Port=2
  wires:
  Pd/1 -> Universal Bridge1/4
  Py/1 -> Universal Bridge/4
  Universal Bridge1/2 -> neg/1
  Universal Bridge1/1 -> Subsystem13/1
  Cd/1 -> Universal Bridge1/3
  Bd/1 -> Universal Bridge1/2
  Ad/1 -> Universal Bridge1/1
  Cy/1 -> Universal Bridge/3
  By/1 -> Universal Bridge/2
  Universal Bridge/1 -> pos/1
  Ay/1 -> Universal Bridge/1
  Universal Bridge/2 -> Subsystem13/Enable

== system case5new/Rectifier/S1 ==
  note: Silvano Casoria
      | Laboratoire simulation de réseaux, IREQ
  From  Workspace : FromWorkspace  VariableName="[T_ramp,  U_ramp]"  SampleTime=0
  Out1 : Outport  InitialOutput=0
  wires:
  From  Workspace/1 -> Out1/1

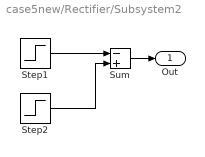
== system case5new/Rectifier/Subsystem2 ==
  Step1 : Step  Time=0.6  After=0.2  SampleTime=0
  Step2 : Step  Time=0.75  After=0.2  SampleTime=0
  Sum : Sum  Inputs=-+  SaturateOnIntegerOverflow=on  InputSameDT=on
  Out : Outport
  wires:
  Sum/1 -> Out/1
  Step2/1 -> Sum/2
  Step1/1 -> Sum/1

== system case5new/Inverter/Measurements/Ia ==
  Out1 : Outport
  wires:
  [tp092417] -> Out1/1

== system case5new/Inverter/Measurements/Ib ==
  Out1 : Outport
  wires:
  [tp092418] -> Out1/1

== system case5new/Inverter/Measurements/Ic ==
  Out1 : Outport
  wires:
  [tp092419] -> Out1/1

== system case5new/Inverter/Measurements/Vb ==
  Out1 : Outport
  wires:
  [tp092415] -> Out1/1

== system case5new/Inverter/Measurements/Vc ==
  Out1 : Outport
  wires:
  [tp092416] -> Out1/1
